simulink subsystem "BatteryMapped"  (R2024a)
settings: Solver=VariableStepAuto  StartTime=0.0  StopTime=10.0  RelTol=1e-3
undefined symbols (not defined in the file): BattAmpHr, BattCurr, BattPwr, BattPwrLoss, BattSoc, BattTemp, BattVolt, PlntBattChrgMax, PlntBattCp, PlntBattMass, PlntBattNumCellSer, PlntBattOpenCirctVolt, PlntBattSocInit, PlntBattTempBpt, PlntBattTempInitDegC, PlntBattVoltSocBpt
libraries: autolibutils x1, autolibdatasheetbattery x1, autolibsharedcommon x1
settings Model: ModifiedByFormat=The MathWorks, Inc.  Creator=The MathWorks, Inc.  LastModifiedBy=The MathWorks, Inc.
settings SolverCC: MaxZcPerStep=1
settings OptimizationCC: ReuseModelBlockBuffer=off
settings DebuggingCC: UnconnectedInputMsg=warning  UnconnectedOutputMsg=warning  UnconnectedLineMsg=warning  SubsystemReferenceDiagnosticForUnitTest=warning
settings ModelReferenceCC: EnableRefExpFcnMdlSchedulingChecks=on
settings RTWCC: GPUComputeCapability=3.5  DLArmComputeVersion=19.05  LargeConstantGeneration=WriteOnlyDNNConstantsToDataFiles

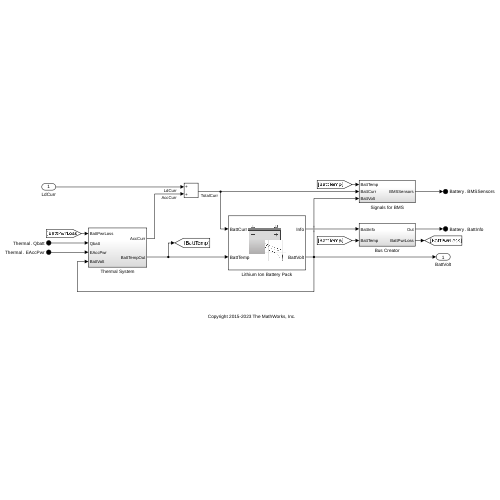
[thumbnail: Simulink's stored preview of the top-level diagram]
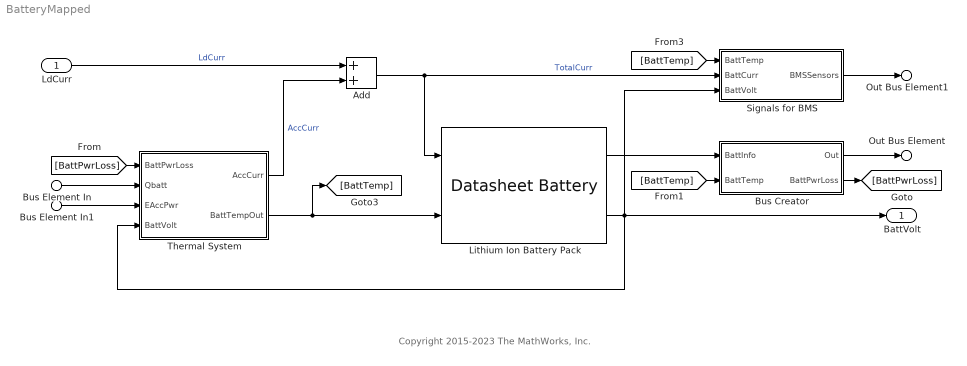
== system BatteryMapped ==
  note: Copyright 2015-2023 The MathWorks, Inc.
  LdCurr : Inport
  Bus Element In : Inport  Port=2  PortName=Thermal  Element=Qbatt
  Bus Element In1 : Inport  Port=2  PortName=Thermal  Element=EAccPwr
  Add : Sum
  Bus Creator : Subsystem
  Lithium Ion Battery Pack : autolibdatasheetbattery/Datasheet Battery  CapacityCtrl=Parameter  OutputVlt=Filtered  BattChargeMax=PlntBattChrgMax  Em=interp2(PlntBattTempBpt,PlntBattVoltSocBpt',PlntBattOpenCirctVolt,PlntBattTempInitDegC,PlntBattVoltSocBpt')'  CapLUTBp=PlntBattVoltSocBpt  RInt=PlntBattIntrnRes'  BattTempBp=PlntBattTempBpt+273.15  CapSOCBp=PlntBattSocBpt  Ns=PlntBattNumCellSer  Np=PlntBattNumCellPar  BattCapInit=PlntBattSocInit*PlntBattChrgMax  Tc=PlntBattTimeCnst  Vinit=interp2(PlntBattTempBpt,PlntBattVoltSocBpt,PlntBattOpenCirctVolt*PlntBattNumCellSer,PlntBattTempInitDegC,PlntBattSocInit)  RefBlkName='autolibdatasheetbattery/Datasheet Battery'
  Signals for BMS : Subsystem
  Thermal System : Subsystem
  BattVolt : Outport  VectorParamsAs1DForOutWhenUnconnected=off
  Out Bus Element : Outport  Port=2  PortName=Battery  Element=BattInfo
  Out Bus Element1 : Outport  Port=2  PortName=Battery  Element=BMSSensors
  wires:
  [BattTemp] -> Bus Creator/2(BattTemp)
  Bus Element In1/1 -> Thermal System/3(EAccPwr)
  Bus Element In/1 -> Thermal System/2(Qbatt)
  [BattPwrLoss] -> Thermal System/1(BattPwrLoss)
  Thermal System/2(BattTempOut) -> Lithium Ion Battery Pack/2, [BattTemp]
  Bus Creator/2(BattPwrLoss) -> [BattPwrLoss]
  Signals for BMS/1(BMSSensors) -> Out Bus Element1/1
  Bus Creator/1(Out) -> Out Bus Element/1
  [BattTemp] -> Signals for BMS/1(BattTemp)
  Lithium Ion Battery Pack/1 -> Bus Creator/1(BattInfo)
  LdCurr/1 -> Add/1  "LdCurr"
  Lithium Ion Battery Pack/2 -> BattVolt/1, Thermal System/4(BattVolt), Signals for BMS/3(BattVolt)
  Thermal System/1(AccCurr) -> Add/2  "AccCurr"
  Add/1 -> Lithium Ion Battery Pack/1, Signals for BMS/2(BattCurr)  "TotalCurr"

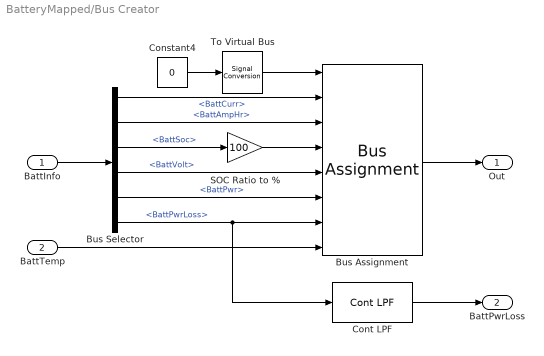
== system BatteryMapped/Bus Creator ==
  BattInfo : Inport
  BattTemp : Inport  Port=2
  Bus Assignment : BusAssignment  AssignedSignals=BattCurr,BattAmpHr,BattSoc,BattVolt,BattPwr,BattPwrLoss,BattTemp
  Bus Selector : BusSelector  OutputSignals=BattCurr,BattAmpHr,BattSoc,BattVolt,BattPwr,BattPwrLoss
  Constant4 : Constant  Value=0  OutDataTypeStr=Bus: BattInfoBUS  SampleTime=Inf
  Cont LPF : autolibutils/Cont LPF  wc=1  AbsoluteTolerance=auto  aMode=6
  SOC Ratio to % : Gain  Gain=100
  To Virtual Bus : SignalConversion  ConversionOutput=Virtual bus  OverrideOpt=off
  Out : Outport
  BattPwrLoss : Outport  Port=2
  wires:
  Cont LPF/1 -> BattPwrLoss/1
  Bus Selector/1 -> Bus Assignment/2  "<BattCurr>"
  SOC Ratio to %/1 -> Bus Assignment/4
  Bus Selector/4 -> Bus Assignment/5  "<BattVolt>"
  To Virtual Bus/1 -> Bus Assignment/1
  Constant4/1 -> To Virtual Bus/1
  BattInfo/1 -> Bus Selector/1
  Bus Selector/3 -> SOC Ratio to %/1  "<BattSoc>"
  Bus Selector/2 -> Bus Assignment/3  "<BattAmpHr>"
  Bus Selector/6 -> Bus Assignment/7, Cont LPF/1  "<BattPwrLoss>"
  Bus Selector/5 -> Bus Assignment/6  "<BattPwr>"
  Bus Assignment/1 -> Out/1
  BattTemp/1 -> Bus Assignment/8

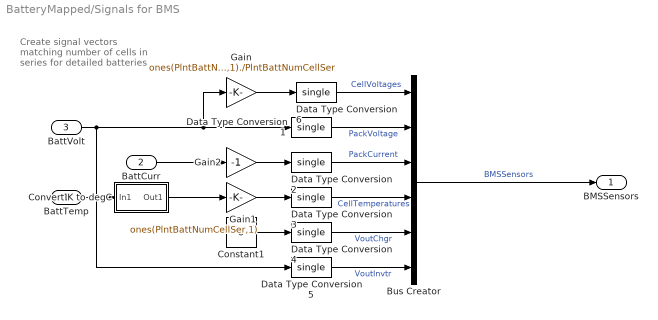
== system BatteryMapped/Signals for BMS ==
  note: Create signal vectors
      | matching number of
      | cells in series for
      | detailed batteries
  BattTemp : Inport
  BattCurr : Inport  Port=2
  BattVolt : Inport  Port=3
  Bus Creator : BusCreator  Inputs=6
  Constant1 : Constant  Value=0
  Convert K to degC : Subsystem
  Data Type Conversion{1..6} (6 alike) : DataTypeConversion  OutDataTypeStr=single  SaturateOnIntegerOverflow=off  RndMeth=Floor
  Gain : Gain  Gain=ones(PlntBattNumCellSer,1)./PlntBattNumCellSer
  Gain1 : Gain  Gain=ones(PlntBattNumCellSer,1)
  Gain2 : Gain  Gain=-1
  BMSSensors : Outport
  wires:
  Bus Creator/1 -> BMSSensors/1  "BMSSensors"
  Data Type Conversion3/1 -> Bus Creator/4  "CellTemperatures"
  Data Type Conversion2/1 -> Bus Creator/3  "PackCurrent"
  Data Type Conversion6/1 -> Bus Creator/1  "CellVoltages"
  Data Type Conversion1/1 -> Bus Creator/2  "PackVoltage"
  Convert K to degC/1(Out1) -> Gain1/1
  Gain2/1 -> Data Type Conversion2/1
  Data Type Conversion5/1 -> Bus Creator/6  "VoutInvtr"
  Gain1/1 -> Data Type Conversion3/1
  Data Type Conversion4/1 -> Bus Creator/5  "VoutChgr"
  BattTemp/1 -> Convert K to degC/1(In1)
  Gain/1 -> Data Type Conversion6/1
  BattVolt/1 -> Data Type Conversion5/1, Gain/1, Data Type Conversion1/1
  Constant1/1 -> Data Type Conversion4/1
  BattCurr/1 -> Gain2/1

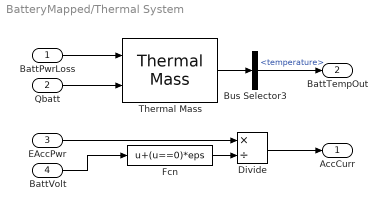
== system BatteryMapped/Thermal System ==
  BattPwrLoss : Inport
  Qbatt : Inport  Port=2
  EAccPwr : Inport  Port=3
  BattVolt : Inport  Port=4
  Bus Selector3 : BusSelector  OutputSignals=temperature
  Divide : Product  Inputs=*/
  Fcn : Fcn  Expr=u+(u==0)*eps
  Thermal Mass : autolibsharedcommon/Thermal Mass  MassOrVol=Mass  Mass=PlntBattMass  Volume=10  Rho=997  HeatCp=PlntBattCp*ones(1,2)  HeatBrkPts=PlntBattCpBpt  Tinit=EnvAirTemp  Tenv=EnvAirTemp  ConvHTC=1  EnvArea=0.1
  AccCurr : Outport
  BattTempOut : Outport  Port=2
  wires:
  BattPwrLoss/1 -> Thermal Mass/1
  Bus Selector3/1 -> BattTempOut/1  "<temperature>"
  Thermal Mass/1 -> Bus Selector3/1
  Qbatt/1 -> Thermal Mass/2
  BattVolt/1 -> Fcn/1
  EAccPwr/1 -> Divide/1
  Divide/1 -> AccCurr/1
  Fcn/1 -> Divide/2

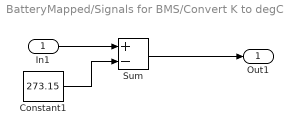
== system BatteryMapped/Signals for BMS/Convert K to degC ==
  In1 : Inport
  Constant1 : Constant  Value=273.15
  Sum : Sum  Inputs=+-
  Out1 : Outport
  wires:
  In1/1 -> Sum/1
  Constant1/1 -> Sum/2
  Sum/1 -> Out1/1
